simulink model "get_descriptor"  (R2015a)
settings: Solver=ode45  StartTime=0.0  StopTime=10.0  RelTol=1e-3
InitFcn:
  | %% DSPBuilder Start
  | alt_dspbuilder_update_model(bdroot)
  | %% DSPBuilder End
libraries: allblocks_alteradspbuilder2 x42
settings Model: Creator=ASUS  LastModifiedBy=ASUS

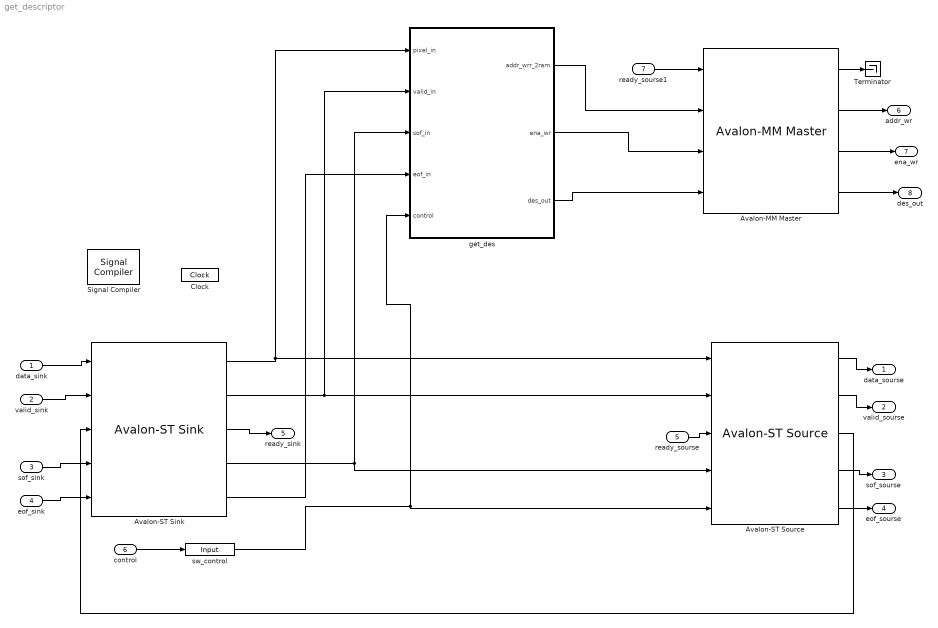
== system get_descriptor ==
  data_sink : Inport
  valid_sink : Inport  Port=2
  sof_sink : Inport  Port=3
  eof_sink : Inport  Port=4
  ready_sourse : Inport  Port=5
  control : Inport  Port=6
  ready_sourse1 : Inport  Port=7
  Avalon-MM Master : allblocks_alteradspbuilder2/Avalon-MM Master  iofile=C:\Users\ASUS\Desktop\final_sift_fpga\tb_get_descriptor\get%5Fdescriptor_Avalon-MM+Master_waitrequest.salt,C:\Users\ASUS\Desktop\final_sift_fpga\tb_get_descriptor\get%5Fdescriptor_Avalon-MM+Master_address.capture,C:\Users\ASUS\Desktop\final_sift_fpga\tb_get_descriptor\get%5Fdescriptor_Avalon-MM+Master_write.capture,C:\Users\ASUS\Desktop\final_sift_fpga\tb_get_descriptor\get%5Fdescriptor_Avalon-MM+Master_writedata.capture,  SpecifyClock=off  addrWidth=32  addrType=Write  BusType=Unsigned Integer  bwl=32  bwr=0  byteEnable=off  flowCtrl=off  pipeline=off  flush=off  burst=off  maxBurst=4  irq=off  irq_mode=Prioritized  externalType=Inferred  PORTTYPE=Input
  Avalon-ST Sink : allblocks_alteradspbuilder2/Avalon-ST Sink  iofile=C:\Users\ASUS\Desktop\final_sift_fpga\tb_get_descriptor\get%5Fdescriptor_Avalon-ST+Sink_data.salt,C:\Users\ASUS\Desktop\final_sift_fpga\tb_get_descriptor\get%5Fdescriptor_Avalon-ST+Sink_valid.salt,C:\Users\ASUS\Desktop\final_sift_fpga\tb_get_descriptor\get%5Fdescriptor_Avalon-ST+Sink_ready.capture,C:\Users\ASUS\Desktop\final_sift_fpga\tb_get_descriptor\get%5Fdescriptor_Avalon-ST+Sink_startofpacket.salt,C:\Users\ASUS\Desktop\final_sift_fpga\tb_get_descriptor\get%5Fdescriptor_Avalon-ST+Sink_endofpacket.salt,  SpecifyClock=off  BusType=Unsigned Integer  bwl=24  bwr=0  symbolWidth=8  symbolsPerBeat=3  numOfChannels=0  numOfErrorDescriptors=0  endOfPacket=on  startOfPacket=on  empty=off  readyLatency=1  externalType=Inferred  PORTTYPE=Output
  Avalon-ST Source : allblocks_alteradspbuilder2/Avalon-ST Source  iofile=C:\Users\ASUS\Desktop\final_sift_fpga\tb_get_descriptor\get%5Fdescriptor_Avalon-ST+Source_data.capture,C:\Users\ASUS\Desktop\final_sift_fpga\tb_get_descriptor\get%5Fdescriptor_Avalon-ST+Source_valid.capture,C:\Users\ASUS\Desktop\final_sift_fpga\tb_get_descriptor\get%5Fdescriptor_Avalon-ST+Source_ready.salt,C:\Users\ASUS\Desktop\final_sift_fpga\tb_get_descriptor\get%5Fdescriptor_Avalon-ST+Source_startofpacket.capture,C:\Users\ASUS\Desktop\final_sift_fpga\tb_get_descriptor\get%5Fdescriptor_Avalon-ST+Source_endofpacket.capture,  SpecifyClock=off  BusType=Unsigned Integer  bwl=24  bwr=0  symbolWidth=8  symbolsPerBeat=3  numOfChannels=0  numOfErrorDescriptors=0  endOfPacket=on  startOfPacket=on  empty=off  readyLatency=1  externalType=Inferred  PORTTYPE=Input
  Clock : allblocks_alteradspbuilder2/Clock  ClockPeriod=10/1.5  ClockPeriodUnit=ns  SampleTime=1  ResetLatency=0  ResetRegisterCascadeDepth=0  SimulationStartCycle=5  PhaseOffset=0  Reset=aclr  ResetType=Active Low  Export=off
  Signal Compiler : allblocks_alteradspbuilder2/Signal Compiler  DeviceFamily=Cyclone IV GX  DeviceName=AUTO  DisableEarlyHDLGeneration=off  EnableSignalTap=off  SignalTapDepth=128  UseBoardBlock=off  StpUseDefaultClock=on  StpClock=Clock  ExportDir=C:\altera\16.0\quartus\dsp_builder  MAX10_ProgrammingMode=Internal Flash (SDM) Single Boot
  Terminator : Terminator
  get_des : Subsystem
  sw_control : allblocks_alteradspbuilder2/Input  iofile=C:\Users\ASUS\Desktop\final_sift_fpga\tb_get_descriptor\get%5Fdescriptor_sw%5Fcontrol.salt  BusType=Unsigned Integer  bwl=18  bwr=0  SpecifyClock=off  PORTTYPE=Input  externalType=Inferred  allowFloatingPointOverride=on  logOutputs=off
  data_sourse : Outport
  valid_sourse : Outport  Port=2
  sof_sourse : Outport  Port=3
  eof_sourse : Outport  Port=4
  ready_sink : Outport  Port=5
  addr_wr : Outport  Port=6
  ena_wr : Outport  Port=7
  des_out : Outport  Port=8
  wires:
  Avalon-ST Sink/1 -> get_des/1(pixel_in), Avalon-ST Source/1
  Avalon-ST Sink/2 -> Avalon-ST Source/2, get_des/2(valid_in)
  Avalon-ST Sink/4 -> get_des/3(sof_in), Avalon-ST Source/4
  sw_control/1 -> Avalon-ST Source/5, get_des/5(control)
  Avalon-ST Sink/5 -> get_des/4(eof_in)
  Avalon-ST Source/3 -> Avalon-ST Sink/3
  Avalon-ST Source/1 -> data_sourse/1
  Avalon-ST Source/2 -> valid_sourse/1
  Avalon-ST Source/4 -> sof_sourse/1
  Avalon-ST Source/5 -> eof_sourse/1
  data_sink/1 -> Avalon-ST Sink/1
  valid_sink/1 -> Avalon-ST Sink/2
  sof_sink/1 -> Avalon-ST Sink/4
  eof_sink/1 -> Avalon-ST Sink/5
  ready_sourse/1 -> Avalon-ST Source/3
  Avalon-ST Sink/3 -> ready_sink/1
  control/1 -> sw_control/1
  get_des/3(des_out) -> Avalon-MM Master/4
  ready_sourse1/1 -> Avalon-MM Master/1
  Avalon-MM Master/1 -> Terminator/1
  get_des/1(addr_wrr_2ram) -> Avalon-MM Master/2
  get_des/2(ena_wr) -> Avalon-MM Master/3
  Avalon-MM Master/2 -> addr_wr/1
  Avalon-MM Master/3 -> ena_wr/1
  Avalon-MM Master/4 -> des_out/1

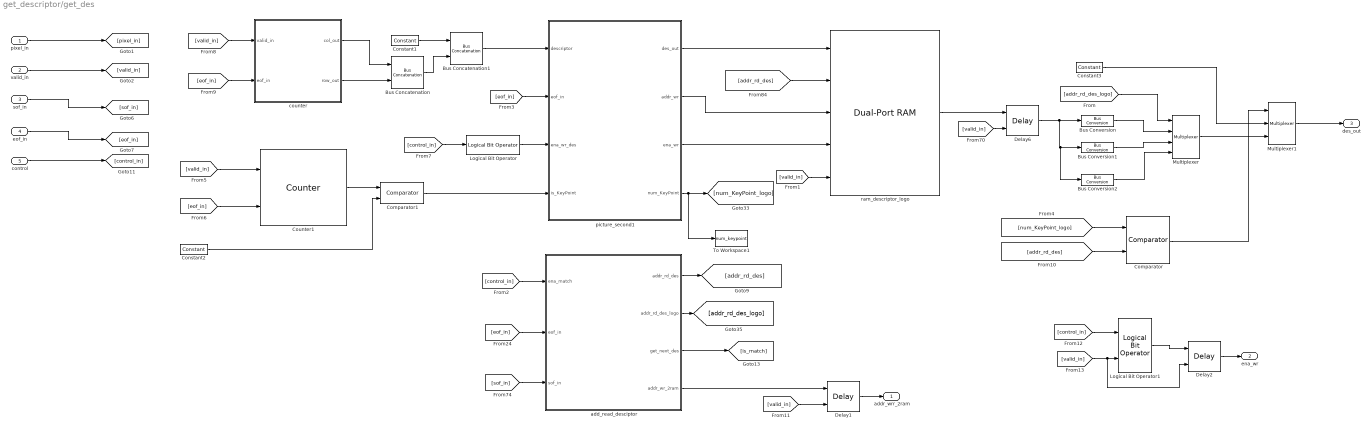
== system get_descriptor/get_des ==
  pixel_in : Inport
  valid_in : Inport  Port=2
  sof_in : Inport  Port=3
  eof_in : Inport  Port=4
  control : Inport  Port=5
  Bus Concatenation : allblocks_alteradspbuilder2/Bus Concatenation  isSigned=off  awidth=32  bwidth=32  pipeline_display=0
  Bus Concatenation1 : allblocks_alteradspbuilder2/Bus Concatenation  isSigned=off  awidth=32  bwidth=64  pipeline_display=0
  Bus Conversion : allblocks_alteradspbuilder2/Bus Conversion  BusType=Unsigned Integer  ibwl=96  ibwr=1  bwl=32  bwr=1  bitToConnectToOutputLSB=64  round=off  saturate=off  pipeline_display=0
  Bus Conversion1 : allblocks_alteradspbuilder2/Bus Conversion  BusType=Unsigned Integer  ibwl=96  ibwr=1  bwl=32  bwr=1  bitToConnectToOutputLSB=32  round=off  saturate=off  pipeline_display=0
  Bus Conversion2 : allblocks_alteradspbuilder2/Bus Conversion  BusType=Unsigned Integer  ibwl=96  ibwr=1  bwl=32  bwr=1  bitToConnectToOutputLSB=0  round=off  saturate=off  pipeline_display=0
  Comparator : allblocks_alteradspbuilder2/Comparator  direction=a >= b  pipeline_display=0  allowFloatingPointOverride=on  logOutputs=off  logFile=C:\Users\ASUS\Desktop\final_sift_fpga\tb_get_descriptor\get%5Fdescriptor_get%5Fdes_Comparator.fixedpointlog
  Comparator1 : allblocks_alteradspbuilder2/Comparator  direction=a == b  pipeline_display=0  allowFloatingPointOverride=on  logOutputs=off  logFile=C:\Users\ASUS\Desktop\final_sift_fpga\tb_get_descriptor\get%5Fdescriptor_get%5Fdes_Comparator1.fixedpointlog
  Constant1 : allblocks_alteradspbuilder2/Constant  mask_cst=1998  BusType=Unsigned Integer  bwl=32  bwr=0  roundMode=Truncate  satMode=Wrap  SpecifyClock=off  allowFloatingPointOverride=on  logOutputs=off  logFile=C:\Users\ASUS\Desktop\final_sift_fpga\tb_get_descriptor\get%5Fdescriptor_get%5Fdes_Constant1.fixedpointlog
  Constant2 : allblocks_alteradspbuilder2/Constant  mask_cst=9999  BusType=Unsigned Integer  bwl=20  bwr=0  roundMode=Truncate  satMode=Wrap  SpecifyClock=off  allowFloatingPointOverride=on  logOutputs=off  logFile=C:\Users\ASUS\Desktop\final_sift_fpga\tb_get_descriptor\get%5Fdescriptor_get%5Fdes_Constant2.fixedpointlog
  Constant3 : allblocks_alteradspbuilder2/Constant  mask_cst=0  BusType=Unsigned Integer  bwl=32  bwr=0  roundMode=Truncate  satMode=Wrap  SpecifyClock=off  allowFloatingPointOverride=on  logOutputs=off  logFile=C:\Users\ASUS\Desktop\final_sift_fpga\tb_get_descriptor\get%5Fdescriptor_get%5Fdes_Constant3.fixedpointlog
  Counter1 : allblocks_alteradspbuilder2/Counter  BusType=Unsigned Integer  bwl=20  bwr=0  use_modulo=on  modulo=10000  SpecifyClock=off  direction=Increment  use_sload=off  use_sset=off  svalue=1  use_clk_ena=off  use_ena=on  use_sclr=on  pipeline_display=1
  Delay1 : allblocks_alteradspbuilder2/Delay  pipeline=3  pipeline_display=3  ClockPhase=1  use_ena=on  use_sclr=off  allowFloatingPointOverride=on  logOutputs=off  logFile=C:\Users\ASUS\Desktop\final_sift_fpga\tb_get_descriptor\get%5Fdescriptor_get%5Fdes_Delay1.fixedpointlog  use_init=off  reset_value=1
  Delay2 : allblocks_alteradspbuilder2/Delay  pipeline=3  pipeline_display=3  ClockPhase=1  use_ena=on  use_sclr=off  allowFloatingPointOverride=on  logOutputs=off  logFile=C:\Users\ASUS\Desktop\final_sift_fpga\tb_get_descriptor\get%5Fdescriptor_get%5Fdes_Delay2.fixedpointlog  use_init=off  reset_value=1
  Delay6 : allblocks_alteradspbuilder2/Delay  pipeline=1  pipeline_display=1  ClockPhase=1  use_ena=on  use_sclr=off  allowFloatingPointOverride=on  logOutputs=off  logFile=C:\Users\ASUS\Desktop\final_sift_fpga\tb_get_descriptor\get%5Fdescriptor_get%5Fdes_Delay6.fixedpointlog  use_init=off  reset_value=1
  Logical Bit Operator : allblocks_alteradspbuilder2/Logical Bit Operator  LogicalOperator=NOT  user_inputs=2  pipeline_display=0
  Logical Bit Operator1 : allblocks_alteradspbuilder2/Logical Bit Operator  LogicalOperator=AND  user_inputs=2  pipeline_display=0
  Multiplexer : allblocks_alteradspbuilder2/Multiplexer  numInputs=3  pipeline=0  oneHot=off  pipeline_display=0  use_ena=off  use_aclr=off  allowFloatingPointOverride=on  logOutputs=off  logFile=C:\Users\ASUS\Desktop\final_sift_fpga\tb_get_descriptor\get%5Fdescriptor_get%5Fdes_Multiplexer.fixedpointlog
  Multiplexer1 : allblocks_alteradspbuilder2/Multiplexer  numInputs=2  pipeline=0  oneHot=off  pipeline_display=0  use_ena=off  use_aclr=off  allowFloatingPointOverride=on  logOutputs=off  logFile=C:\Users\ASUS\Desktop\final_sift_fpga\tb_get_descriptor\get%5Fdescriptor_get%5Fdes_Multiplexer1.fixedpointlog
  To Workspace1 : ToWorkspace  VariableName=num_keypoint  SaveFormat=Timeseries  SampleTime=-1
  add_read_desciptor : Subsystem
  counter : Subsystem
  picture_second1 : Subsystem
  ram_descriptor_logo : allblocks_alteradspbuilder2/Dual-Port RAM  numwords=100  BusType=Unsigned Integer  bwl=96  bwr=0  memory_type=AUTO  ram_type=DualRAM  dont_care=on  initialization=Blank  init_file=input.hex  init_array=[0:1:15]  register_outputs=on  use_ena=on  ClockPhase=1  allowFloatingPointOverride=on  logOutputs=off  logFile=C:\Users\ASUS\Desktop\final_sift_fpga\tb_get_descriptor\get%5Fdescriptor_get%5Fdes_ram%5Fdescriptor%5Flogo.fixedpointlog  pipeline_display=2
  addr_wrr_2ram : Outport
  ena_wr : Outport  Port=2
  des_out : Outport  Port=3
  wires:
  valid_in/1 -> [valid_in]
  sof_in/1 -> [sof_in]
  pixel_in/1 -> [pixel_in]
  eof_in/1 -> [eof_in]
  control/1 -> [control_in]
  picture_second1/2(addr_wr) -> ram_descriptor_logo/3
  picture_second1/4(num_KeyPoint) -> To Workspace1/1, [num_KeyPoint_logo]
  Delay6/1 -> Bus Conversion2/1, Bus Conversion1/1, Bus Conversion/1
  [valid_in] -> Delay6/2
  [eof_in] -> picture_second1/2(eof_in)
  picture_second1/3(ena_wr) -> ram_descriptor_logo/4
  [valid_in] -> counter/1(valid_in)
  [eof_in] -> counter/2(eof_in)
  Bus Concatenation1/1 -> picture_second1/1(descriptor)
  ram_descriptor_logo/1 -> Delay6/1
  [addr_rd_des] -> ram_descriptor_logo/2
  picture_second1/1(des_out) -> ram_descriptor_logo/1
  [eof_in] -> add_read_desciptor/2(eof_in)
  add_read_desciptor/3(get_next_des) -> [is_match]
  Constant2/1 -> Comparator1/2
  [sof_in] -> add_read_desciptor/3(sof_in)
  Bus Concatenation/1 -> Bus Concatenation1/2
  [addr_rd_des_logo] -> Multiplexer/1
  [valid_in] -> ram_descriptor_logo/5
  [num_KeyPoint_logo] -> Comparator/1
  counter/2(row_out) -> Bus Concatenation/2
  add_read_desciptor/2(addr_rd_des_logo) -> [addr_rd_des_logo]
  Multiplexer1/1 -> des_out/1
  Counter1/1 -> Comparator1/1
  Comparator1/1 -> picture_second1/4(is_KeyPoint)
  [eof_in] -> Counter1/2
  [control_in] -> Logical Bit Operator/1
  add_read_desciptor/1(addr_rd_des) -> [addr_rd_des]
  Logical Bit Operator/1 -> picture_second1/3(ena_wr_des)
  Multiplexer/1 -> Multiplexer1/3
  Bus Conversion2/1 -> Multiplexer/4
  [control_in] -> add_read_desciptor/1(ena_match)
  Bus Conversion/1 -> Multiplexer/2
  Constant3/1 -> Multiplexer1/2
  counter/1(col_out) -> Bus Concatenation/1
  [addr_rd_des] -> Comparator/2
  Constant1/1 -> Bus Concatenation1/1
  [valid_in] -> Counter1/1
  Comparator/1 -> Multiplexer1/1
  Bus Conversion1/1 -> Multiplexer/3
  add_read_desciptor/4(addr_wr_2ram) -> Delay1/1
  [valid_in] -> Delay1/2
  Delay1/1 -> addr_wrr_2ram/1
  [control_in] -> Logical Bit Operator1/1
  [valid_in] -> Delay2/2, Logical Bit Operator1/2
  Logical Bit Operator1/1 -> Delay2/1
  Delay2/1 -> ena_wr/1

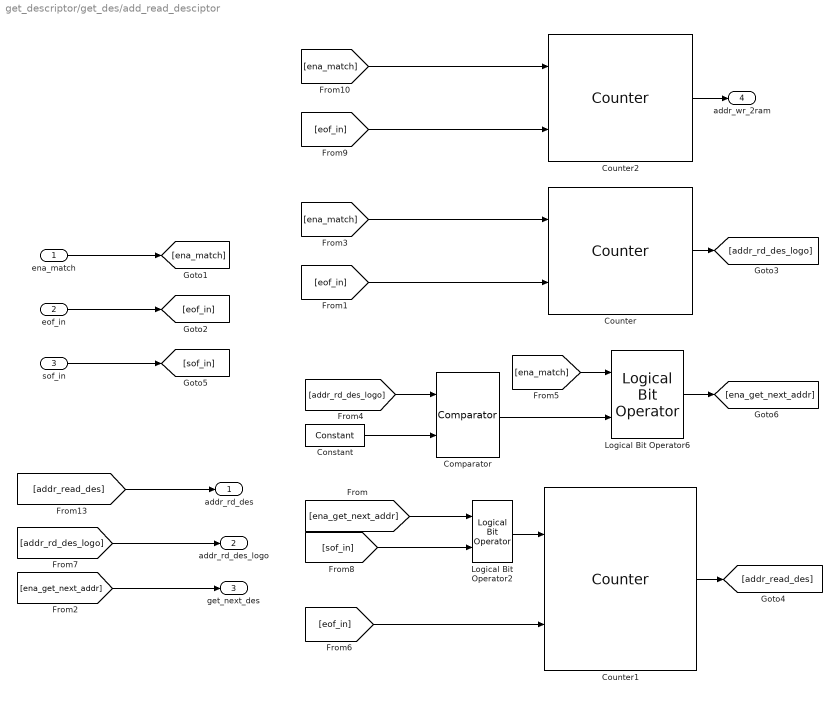
== system get_descriptor/get_des/add_read_desciptor ==
  ena_match : Inport
  eof_in : Inport  Port=2
  sof_in : Inport  Port=3
  Comparator : allblocks_alteradspbuilder2/Comparator  direction=a == b  pipeline_display=0  allowFloatingPointOverride=on  logOutputs=off  logFile=C:\Users\ASUS\Desktop\final_sift_fpga\tb_get_descriptor\get%5Fdescriptor_get%5Fdes_add%5Fread%5Fdesciptor_Comparator.fixedpointlog
  Constant : allblocks_alteradspbuilder2/Constant  mask_cst=2  BusType=Unsigned Integer  bwl=2  bwr=0  roundMode=Truncate  satMode=Wrap  SpecifyClock=off  allowFloatingPointOverride=on  logOutputs=off  logFile=C:\Users\ASUS\Desktop\final_sift_fpga\tb_get_descriptor\get%5Fdescriptor_get%5Fdes_add%5Fread%5Fdesciptor_Constant.fixedpointlog
  Counter : allblocks_alteradspbuilder2/Counter  BusType=Unsigned Integer  bwl=2  bwr=0  use_modulo=on  modulo=3  SpecifyClock=off  direction=Increment  use_sload=off  use_sset=off  svalue=1  use_clk_ena=off  use_ena=on  use_sclr=on  pipeline_display=1
  Counter1 : allblocks_alteradspbuilder2/Counter  BusType=Unsigned Integer  bwl=7  bwr=0  use_modulo=on  modulo=100  SpecifyClock=off  direction=Increment  use_sload=off  use_sset=off  svalue=0  use_clk_ena=off  use_ena=on  use_sclr=on  pipeline_display=1
  Counter2 : allblocks_alteradspbuilder2/Counter  BusType=Unsigned Integer  bwl=9  bwr=0  use_modulo=on  modulo=300  SpecifyClock=off  direction=Increment  use_sload=off  use_sset=off  svalue=1  use_clk_ena=off  use_ena=on  use_sclr=on  pipeline_display=1
  Logical Bit Operator2 : allblocks_alteradspbuilder2/Logical Bit Operator  LogicalOperator=OR  user_inputs=2  pipeline_display=0
  Logical Bit Operator6 : allblocks_alteradspbuilder2/Logical Bit Operator  LogicalOperator=AND  user_inputs=2  pipeline_display=0
  addr_rd_des : Outport
  addr_rd_des_logo : Outport  Port=2
  get_next_des : Outport  Port=3
  addr_wr_2ram : Outport  Port=4
  wires:
  [addr_rd_des_logo] -> Comparator/1
  ena_match/1 -> [ena_match]
  Constant/1 -> Comparator/2
  Counter1/1 -> [addr_read_des]
  Counter/1 -> [addr_rd_des_logo]
  [addr_read_des] -> addr_rd_des/1
  Comparator/1 -> Logical Bit Operator6/2
  [ena_match] -> Counter/1
  Logical Bit Operator6/1 -> [ena_get_next_addr]
  eof_in/1 -> [eof_in]
  [eof_in] -> Counter/2
  [ena_match] -> Logical Bit Operator6/1
  [ena_get_next_addr] -> get_next_des/1
  [eof_in] -> Counter1/2
  [ena_get_next_addr] -> Logical Bit Operator2/1
  sof_in/1 -> [sof_in]
  Logical Bit Operator2/1 -> Counter1/1
  [sof_in] -> Logical Bit Operator2/2
  [addr_rd_des_logo] -> addr_rd_des_logo/1
  Counter2/1 -> addr_wr_2ram/1
  [ena_match] -> Counter2/1
  [eof_in] -> Counter2/2

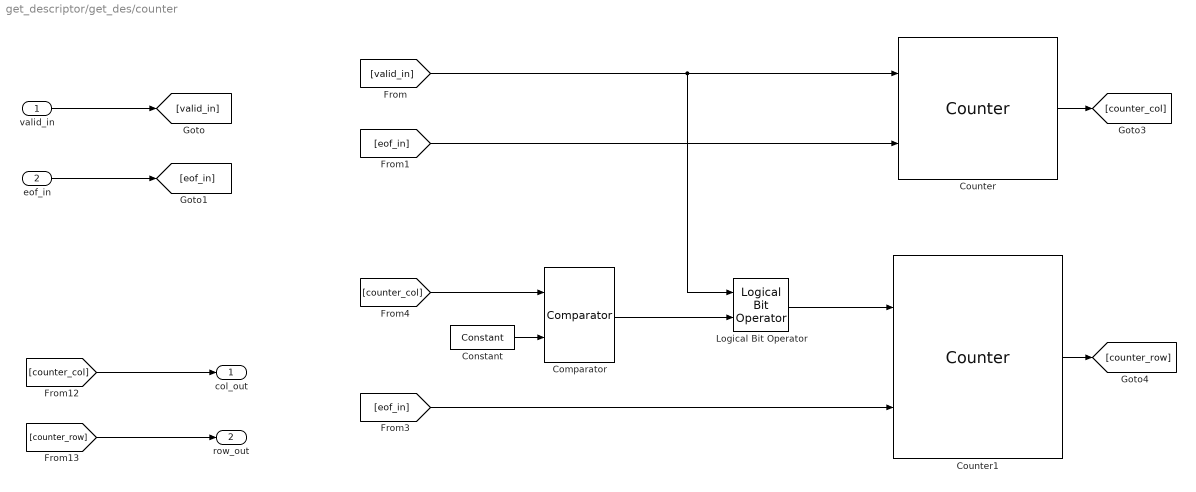
== system get_descriptor/get_des/counter ==
  valid_in : Inport
  eof_in : Inport  Port=2
  Comparator : allblocks_alteradspbuilder2/Comparator  direction=a == b  pipeline_display=0  allowFloatingPointOverride=on  logOutputs=off  logFile=C:\Users\ASUS\Desktop\final_sift_fpga\tb_get_descriptor\get%5Fdescriptor_get%5Fdes_counter_Comparator.fixedpointlog
  Constant : allblocks_alteradspbuilder2/Constant  mask_cst=639  BusType=Unsigned Integer  bwl=10  bwr=0  roundMode=Truncate  satMode=Wrap  SpecifyClock=off  allowFloatingPointOverride=on  logOutputs=off  logFile=C:\Users\ASUS\Desktop\final_sift_fpga\tb_get_descriptor\get%5Fdescriptor_get%5Fdes_counter_Constant.fixedpointlog
  Counter : allblocks_alteradspbuilder2/Counter  BusType=Unsigned Integer  bwl=10  bwr=0  use_modulo=on  modulo=640  SpecifyClock=off  direction=Increment  use_sload=off  use_sset=off  svalue=1  use_clk_ena=off  use_ena=on  use_sclr=on  pipeline_display=1
  Counter1 : allblocks_alteradspbuilder2/Counter  BusType=Unsigned Integer  bwl=10  bwr=0  use_modulo=on  modulo=480  SpecifyClock=off  direction=Increment  use_sload=off  use_sset=off  svalue=0  use_clk_ena=off  use_ena=on  use_sclr=on  pipeline_display=1
  Logical Bit Operator : allblocks_alteradspbuilder2/Logical Bit Operator  LogicalOperator=AND  user_inputs=2  pipeline_display=0
  col_out : Outport
  row_out : Outport  Port=2
  wires:
  [eof_in] -> Counter1/2
  Logical Bit Operator/1 -> Counter1/1
  [counter_col] -> Comparator/1
  eof_in/1 -> [eof_in]
  Constant/1 -> Comparator/2
  Comparator/1 -> Logical Bit Operator/2
  valid_in/1 -> [valid_in]
  Counter1/1 -> [counter_row]
  Counter/1 -> [counter_col]
  [valid_in] -> Logical Bit Operator/1, Counter/1
  [counter_row] -> row_out/1
  [counter_col] -> col_out/1
  [eof_in] -> Counter/2

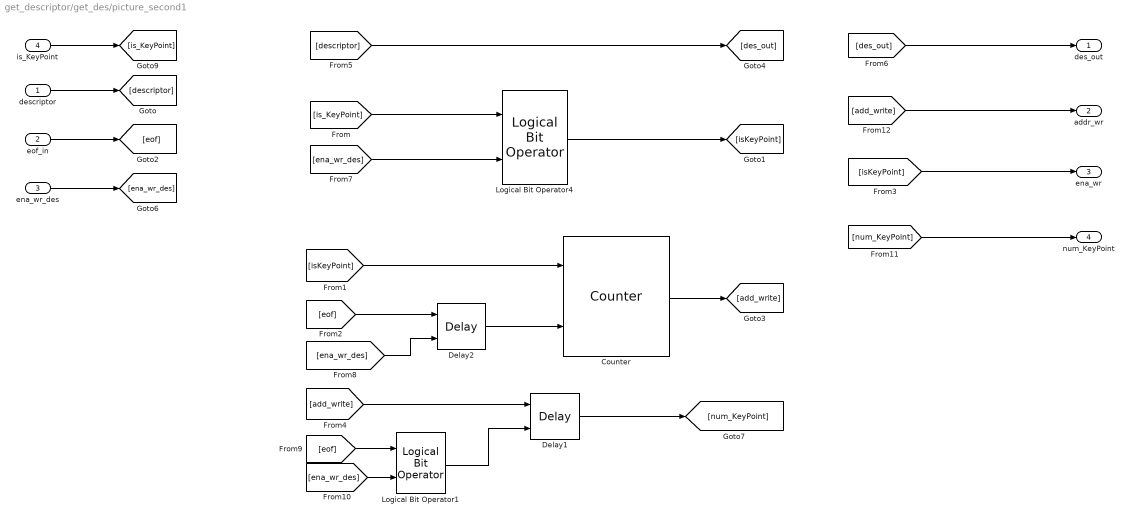
== system get_descriptor/get_des/picture_second1 ==
  descriptor : Inport
  eof_in : Inport  Port=2
  ena_wr_des : Inport  Port=3
  is_KeyPoint : Inport  Port=4
  Counter : allblocks_alteradspbuilder2/Counter  BusType=Unsigned Integer  bwl=7  bwr=0  use_modulo=on  modulo=100  SpecifyClock=off  direction=Increment  use_sload=off  use_sset=off  svalue=1  use_clk_ena=off  use_ena=on  use_sclr=on  pipeline_display=1
  Delay1 : allblocks_alteradspbuilder2/Delay  pipeline=1  pipeline_display=1  ClockPhase=1  use_ena=on  use_sclr=off  allowFloatingPointOverride=on  logOutputs=off  logFile=C:\Users\ASUS\Desktop\final_sift_fpga\tb_get_descriptor\get%5Fdescriptor_get%5Fdes_picture%5Fsecond1_Delay1.fixedpointlog  use_init=off  reset_value=1
  Delay2 : allblocks_alteradspbuilder2/Delay  pipeline=5  pipeline_display=5  ClockPhase=1  use_ena=on  use_sclr=off  allowFloatingPointOverride=on  logOutputs=off  logFile=C:\Users\ASUS\Desktop\final_sift_fpga\tb_get_descriptor\get%5Fdescriptor_get%5Fdes_picture%5Fsecond1_Delay2.fixedpointlog  use_init=off  reset_value=1
  Logical Bit Operator1 : allblocks_alteradspbuilder2/Logical Bit Operator  LogicalOperator=AND  user_inputs=2  pipeline_display=0
  Logical Bit Operator4 : allblocks_alteradspbuilder2/Logical Bit Operator  LogicalOperator=AND  user_inputs=2  pipeline_display=0
  des_out : Outport
  addr_wr : Outport  Port=2
  ena_wr : Outport  Port=3
  num_KeyPoint : Outport  Port=4
  wires:
  descriptor/1 -> [descriptor]
  eof_in/1 -> [eof]
  ena_wr_des/1 -> [ena_wr_des]
  Counter/1 -> [add_write]
  [descriptor] -> [des_out]
  [isKeyPoint] -> Counter/1
  [des_out] -> des_out/1
  [add_write] -> addr_wr/1
  [isKeyPoint] -> ena_wr/1
  [is_KeyPoint] -> Logical Bit Operator4/1
  Logical Bit Operator4/1 -> [isKeyPoint]
  [ena_wr_des] -> Logical Bit Operator4/2
  Delay1/1 -> [num_KeyPoint]
  [num_KeyPoint] -> num_KeyPoint/1
  is_KeyPoint/1 -> [is_KeyPoint]
  [eof] -> Delay2/1
  [add_write] -> Delay1/1
  Delay2/1 -> Counter/2
  [ena_wr_des] -> Delay2/2
  [eof] -> Logical Bit Operator1/1
  [ena_wr_des] -> Logical Bit Operator1/2
  Logical Bit Operator1/1 -> Delay1/2
